simulink model "Ryzhii14"  (R2023b)
settings: Solver=VariableStepAuto  StartTime=0.0  StopTime=t(end)  RelTol=1e-3
values from neighbouring files (symbols this model uses):
  params = [ ... (first row only)    [gois09_simulink.m]    (also in ryzhii14_simulink.m; sinoatrial_simulink.m; vdp_simulink.m)
  xInitial = [initial_conditions ... (first row only)    [gois09_simulink.m]    (also in hilaire07martinez_simulink.m = initial_conditions(1:2); jewett99_simulink.m = initial_conditions(1:2); ryzhii14_simulink.m; sinoatrial_simulink.m = initial_conditions)
settings Model: Creator=chukw  LastModifiedBy=chukw

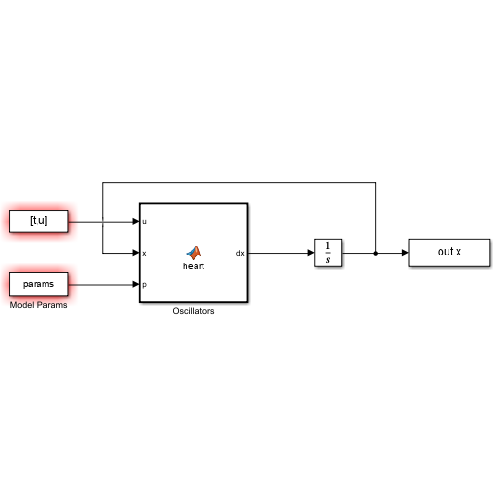
[thumbnail: Simulink's stored preview of the top-level diagram]
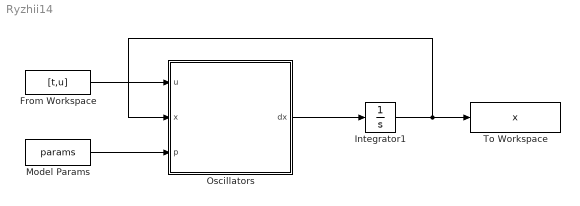
== system Ryzhii14 ==
  From Workspace : FromWorkspace  VariableName=[t,u]
  Integrator1 : Integrator  InitialCondition=xInitial
  Model Params : Constant  Value=params
  Oscillators : MATLAB Function  TreatAsAtomicUnit=on
  To Workspace : ToWorkspace  VariableName=x  SampleTime=-1
  wires:
  Model Params/1 -> Oscillators/3(p)
  From Workspace/1 -> Oscillators/1(u)
  Oscillators/1(dx) -> Integrator1/1
  Integrator1/1 -> Oscillators/2(x), To Workspace/1

== matlab function Ryzhii14/Oscillators ==
  data: u input; dx output; x input; p input
function dx = heart(u, x, p)
    a1 = p(1);
    u11 = p(2);
    u12 = p(3);
    f1 = p(4);
    d1 = p(5);
    e1 = p(6);

    % AV Node.
    a2 = p(7);
    u21 = p(8);
    u22 = p(9);
    f2 = p(10);
    d2 = p(11);
    e2 = p(12);

    % HP Complex.
    a3 = p(13);
    u31 = p(14);
    u32 = p(15);
    f3 = p(16);
    d3 = p(17);
    e3 = p(18);

    % Coupling Params.
    k_sa_av = p(19);
    k_av_hp = p(20);

    % ECG Params;
    alf_0 = p(21);
    alf_1 = p(22);
    alf_3 = p(23);
    alf_5 = p(24);

    % Differential equations.
    dx = zeros(7, 1);

    % SA Node.
    dx(1) = x(2);
    dx(2) = (-a1*x(2)*(x(1) - u11)*(x(1) - u12)) -...
        (f1*x(1)*(x(1) + d1)*(x(1) + e1));

    % AV Node.
    dx(3) = x(4);
    dx(4) = (-a2*x(4)*(x(3) - u21)*(x(3) - u22)) -...
        (f2*x(3)*(x(3) + d2)*(x(3) + e2)) +...
        (k_sa_av*(x(2) - x(4)));

    % HP Complex.
    dx(5) = x(6);
    dx(6) = (-a3*x(6)*(x(5) - u31)*(x(5) - u32)) -...
        (f3*x(5)*(x(5) + d3)*(x(5) + e3)) +...
        (k_av_hp*(x(4) - x(6)));

    % ECG.
    dx(7) = (alf_1*x(2)) + (alf_3*x(4)) + (alf_5*x(6));
end
